simulink model "LongitudinalVehicle"  (R2020a)
settings: Solver=FixedStepDiscrete  StartTime=0.0  StopTime=10.0  FixedStep=0.01  RelTol=1e-3
undefined symbols (not defined in the file or in its folder): D_VEH_INIT_SPD, DiscIntNeverNeededParam
settings Model: Creator=ddaiy  LastModifiedBy=ddaiy
settings DataIOCC: InspectSignalLogs=on
settings DebuggingCC: SignalRangeChecking=warning  SignalResolutionControl=TryResolveAllWithWarning  IntegerOverflowMsg=error  ParameterUnderflowMsg=error  ParameterPrecisionLossMsg=none  UnderSpecifiedDataTypeMsg=error  UnnecessaryDatatypeConvMsg=warning  SignalLabelMismatchMsg=error  UnconnectedInputMsg=error  UnconnectedOutputMsg=error  UnconnectedLineMsg=error  BusObjectLabelMismatch=error  ModelReferenceIOMsg=error  ModelReferenceVersionMismatchMessage=error  ModelReferenceIOMismatchMessage=error  StrictBusMsg=WarnOnBusTreatedAsVector  NonBusSignalsTreatedAsBus=warning  IntegerSaturationMsg=error  UnderSpecifiedDimensionMsg=error
settings ModelReferenceCC: ModelReferenceNumInstancesAllowed=Single

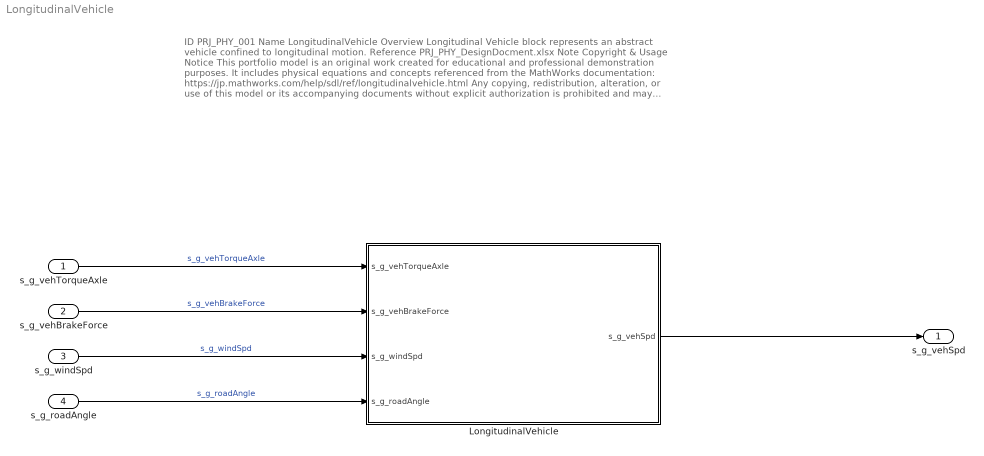
== system LongitudinalVehicle ==
  note: ID
      | PRJ_PHY_001
      |
      | Name
      | LongitudinalVehicle
      |
      | Overview
      | Longitudinal Vehicle block represents an abstract vehicle confined to longitudinal motion.
      |
      | Reference
      | ​PRJ_PHY_DesignDocment.xlsx
      |
      | Note
      | ​Copyright & Usage Notice
      | This portfolio model is an original work created for educational and professional demonstration purposes.
      | It includes physical equations and concepts referenced from the MathWorks documentation:
      | https://jp.mathworks.com/help/sdl/ref/longitudinalvehicle.html
      | Any copying, redistribution, alteration, or use of this model or its accompanying documents without explicit authorization is prohibited and may violate applicable intellectual property laws.
  s_g_vehTorqueAxle : Inport  Description=torque at axle  OutDataTypeStr=single  PortDimensions=1
      settings: AttributesFormatString=%<Description>
  s_g_vehBrakeForce : Inport  Description=brake force input  Port=2  OutDataTypeStr=single  PortDimensions=1
      settings: AttributesFormatString=%<Description>
  s_g_windSpd : Inport  Description=longitudinal wind speed.  Port=3  OutDataTypeStr=single  PortDimensions=1
      settings: AttributesFormatString=%<Description>
  s_g_roadAngle : Inport  Description=road incline angle input  Port=4  OutDataTypeStr=single  PortDimensions=1
      settings: AttributesFormatString=%<Description>
  LongitudinalVehicle : Subsystem  Description=Longitudinal Vehicle block represents an abstract vehicle confined to longitudinal motion.
      settings: AttributesFormatString=%<Description>
  s_g_vehSpd : Outport  Description=longitudinal velocity output  PortDimensions=1
      settings: AttributesFormatString=%<Description>
  wires:
  s_g_vehBrakeForce/1 -> LongitudinalVehicle/2(s_g_vehBrakeForce)  "s_g_vehBrakeForce"
  s_g_vehTorqueAxle/1 -> LongitudinalVehicle/1(s_g_vehTorqueAxle)  "s_g_vehTorqueAxle"
  s_g_windSpd/1 -> LongitudinalVehicle/3(s_g_windSpd)  "s_g_windSpd"
  s_g_roadAngle/1 -> LongitudinalVehicle/4(s_g_roadAngle)  "s_g_roadAngle"
  LongitudinalVehicle/1(s_g_vehSpd) -> s_g_vehSpd/1

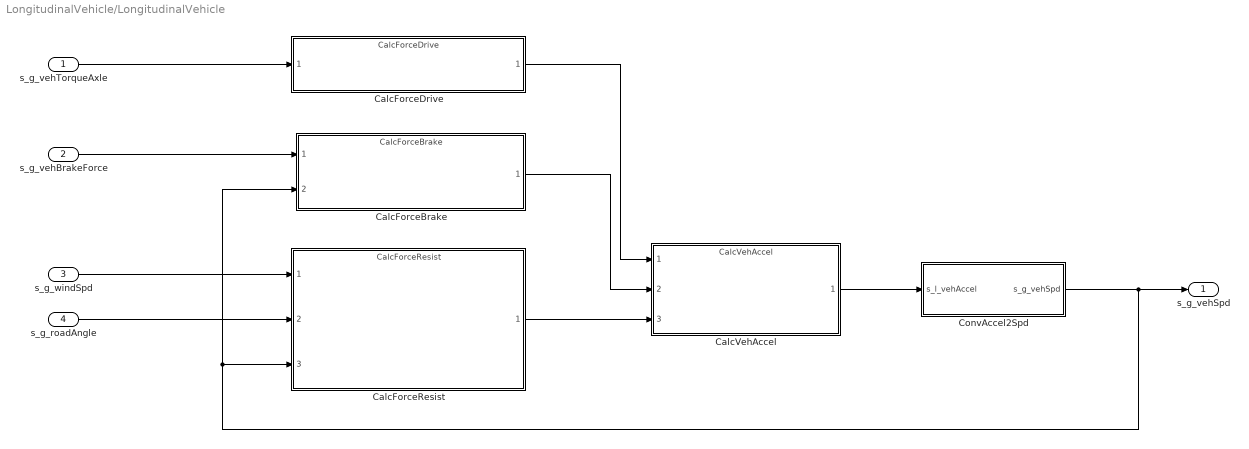
== system LongitudinalVehicle/LongitudinalVehicle ==
  s_g_vehTorqueAxle : Inport  Description=torque at axle
      settings: AttributesFormatString=%<Description>
  s_g_vehBrakeForce : Inport  Description=brake force input  Port=2
      settings: AttributesFormatString=%<Description>
  s_g_windSpd : Inport  Description=longitudinal wind speed.  Port=3
      settings: AttributesFormatString=%<Description>
  s_g_roadAngle : Inport  Description=road incline angle input  Port=4
      settings: AttributesFormatString=%<Description>
  CalcForceBrake : ModelReference  Description=PRJ_PHY_001_002  ModelNameDialog=CalcForceBrake  ModelReferenceVersion=1.11
      settings: AttributesFormatString=%<Description>
  CalcForceDrive : ModelReference  Description=PRJ_PHY_001_001  ModelNameDialog=CalcForceDrive  ModelReferenceVersion=1.8
      settings: AttributesFormatString=%<Description>
  CalcForceResist : ModelReference  Description=PRJ_PHY_001_003  ModelNameDialog=CalcForceResist  ModelReferenceVersion=1.11
      settings: AttributesFormatString=%<Description>
  CalcVehAccel : ModelReference  Description=PRJ_PHY_001_004  ModelNameDialog=CalcVehAccel.slx  ModelReferenceVersion=1.11
      settings: AttributesFormatString=%<Description>
  ConvAccel2Spd : Subsystem
  s_g_vehSpd : Outport  Description=longitudinal velocity output
      settings: AttributesFormatString=%<Description>
  wires:
  CalcForceResist/1 -> CalcVehAccel/3
  CalcForceBrake/1 -> CalcVehAccel/2
  CalcForceDrive/1 -> CalcVehAccel/1
  s_g_vehTorqueAxle/1 -> CalcForceDrive/1
  s_g_vehBrakeForce/1 -> CalcForceBrake/1
  s_g_windSpd/1 -> CalcForceResist/1
  s_g_roadAngle/1 -> CalcForceResist/2
  ConvAccel2Spd/1(s_g_vehSpd) -> CalcForceBrake/2, CalcForceResist/3, s_g_vehSpd/1
  CalcVehAccel/1 -> ConvAccel2Spd/1(s_l_vehAccel)

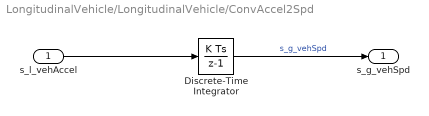
== system LongitudinalVehicle/LongitudinalVehicle/ConvAccel2Spd ==
  s_l_vehAccel : Inport  Description=longitudinal accel
      settings: AttributesFormatString=%<Description>
  Discrete-Time Integrator : DiscreteIntegrator  InitialCondition=D_VEH_INIT_SPD  SampleTime=-1  ICPrevOutput=DiscIntNeverNeededParam  ICPrevScaledInput=DiscIntNeverNeededParam
  s_g_vehSpd : Outport  Description=longitudinal velocity output
      settings: AttributesFormatString=%<Description>
  wires:
  Discrete-Time Integrator/1 -> s_g_vehSpd/1  "s_g_vehSpd"
  s_l_vehAccel/1 -> Discrete-Time Integrator/1
